simulink model "bfsk_demodulation_ber"  (R2021a)
settings: Solver=VariableStepAuto  StartTime=0.0  StopTime=2  RelTol=1e-3
libraries: dspsrcs4 x6, commfilt2 x5, commsink2 x2, commchan3 x1, commanapbnd3 x1, commrandsrc3 x1, simulink x1
settings Model: Creator=joycelai  LastModifiedBy=joycelai

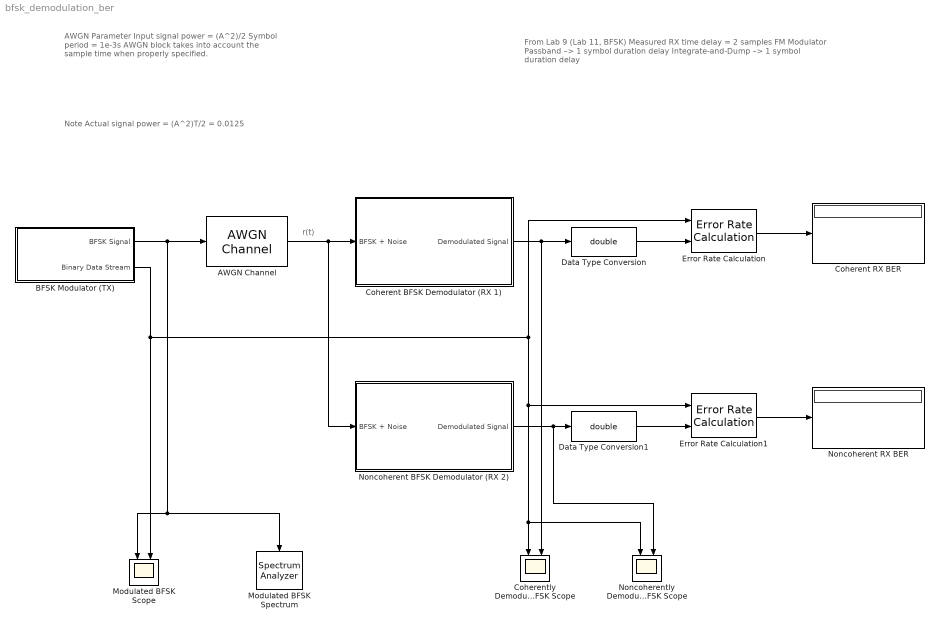
== system bfsk_demodulation_ber ==
  note: AWGN Parameter
      | Input signal power = (A^2)/2
      | Symbol period = 1e-3s
      |
      | AWGN block takes into account the
      | sample time when properly specified.
  note: r(t)
  note: Note
      | Actual signal power = (A^2)T/2 = 0.0125
  note: From Lab 9 (Lab 11, BFSK)
      | Measured RX time delay = 2 samples
      |
      | FM Modulator Passband –> 1 symbol duration delay
      | Integrate-and-Dump –> 1 symbol duration delay
  AWGN Channel : commchan3/AWGN Channel  InputProcessing=Columns as channels (frame based)  seed=67  noiseMode="Signal to noise ratio  (Eb/No)"  EbNodB=2  EsNodB=10  SNRdB=10  bitsPerSym=1  Ps=25/2  Tsym=1e-3  variance=1
  BFSK Modulator (TX) : Subsystem
  Coherent BFSK Demodulator (RX 1) : Subsystem
  Coherent RX BER : Display
      settings: Decimation=14
  Coherently Demodulated BFSK Scope : Scope  NumInputPorts=2
  Data Type Conversion : DataTypeConversion  OutDataTypeStr=double
  Data Type Conversion1 : DataTypeConversion  OutDataTypeStr=double
  Error Rate Calculation : commsink2/Error Rate Calculation  N=2  st_delay=0  cp_mode=Entire frame  subframe=[]  PMode=Port  WsName=ErrorVec  RsMode2=off  stop=off  numErr=100  maxBits=1e6
  Error Rate Calculation1 : commsink2/Error Rate Calculation  N=2  st_delay=0  cp_mode=Entire frame  subframe=[]  PMode=Port  WsName=ErrorVec  RsMode2=off  stop=off  numErr=100  maxBits=1e6
  Modulated BFSK Scope : Scope  NumInputPorts=2
  Modulated BFSK Spectrum : SpectrumAnalyzer
  Noncoherent BFSK Demodulator (RX 2) : Subsystem
  Noncoherent RX BER : Display
      settings: Decimation=14
  Noncoherently Demodulated BFSK Scope : Scope  NumInputPorts=2
  wires:
  Data Type Conversion/1 -> Error Rate Calculation/2
  BFSK Modulator (TX)/1(BFSK Signal) -> AWGN Channel/1, Modulated BFSK Spectrum/1, Modulated BFSK Scope/1
  Coherent BFSK Demodulator (RX 1)/1(Demodulated Signal) -> Data Type Conversion/1, Coherently Demodulated BFSK Scope/2
  BFSK Modulator (TX)/2(Binary Data Stream) -> Modulated BFSK Scope/2, Noncoherently Demodulated BFSK Scope/1, Coherently Demodulated BFSK Scope/1, Error Rate Calculation1/1, Error Rate Calculation/1
  Error Rate Calculation/1 -> Coherent RX BER/1
  AWGN Channel/1 -> Noncoherent BFSK Demodulator (RX 2)/1(BFSK + Noise), Coherent BFSK Demodulator (RX 1)/1(BFSK + Noise)
  Error Rate Calculation1/1 -> Noncoherent RX BER/1
  Data Type Conversion1/1 -> Error Rate Calculation1/2
  Noncoherent BFSK Demodulator (RX 2)/1(Demodulated Signal) -> Noncoherently Demodulated BFSK Scope/2, Data Type Conversion1/1

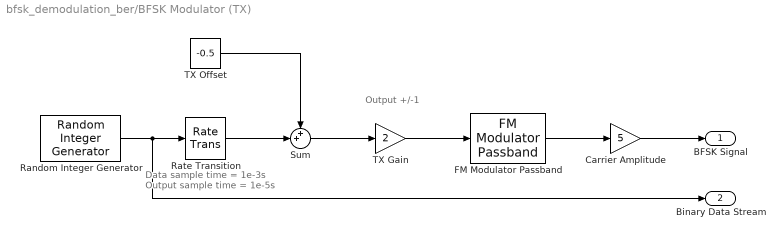
== system bfsk_demodulation_ber/BFSK Modulator (TX) ==
  note: Data sample time = 1e-3s
      | Output sample time = 1e-5s
  note: Output +/-1
  Carrier Amplitude : Gain  Gain=5
  FM Modulator Passband : commanapbnd3/FM Modulator Passband  Fc=10e3  Ph=pi/10  Kc=3e3
      settings: SourceProductBaseCode=CM
  Random Integer Generator : commrandsrc3/Random Integer Generator  SetSize=2  SeedSource=Auto  Seed=0  SampleTime=1e-3  SamplesPerFrame=1  OutputDataType=double  SimulateUsing=Interpreted execution
  Rate Transition : RateTransition  OutPortSampleTime=1e-5
  Sum : Sum  Inputs=++|
  TX Gain : Gain  Gain=2
  TX Offset : Constant  Value=-0.5
  BFSK Signal : Outport
  Binary Data Stream : Outport  Port=2
  wires:
  Random Integer Generator/1 -> Binary Data Stream/1, Rate Transition/1
  TX Gain/1 -> FM Modulator Passband/1
  Sum/1 -> TX Gain/1
  Carrier Amplitude/1 -> BFSK Signal/1
  FM Modulator Passband/1 -> Carrier Amplitude/1
  TX Offset/1 -> Sum/1
  Rate Transition/1 -> Sum/2

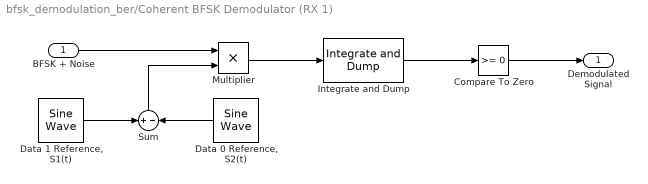
== system bfsk_demodulation_ber/Coherent BFSK Demodulator (RX 1) ==
  BFSK + Noise : Inport
  Compare To Zero : simulink/Logic and Bit Operations/Compare To Zero  relop=>=  OutDataTypeStr=uint8
  "Data 0 Reference, S2(t)" : dspsrcs4/Sine Wave  Amplitude=1  Frequency=(10e3)-(3e3)  Phase=pi/2+pi/10  SampleMode=Discrete  OutComplex=Real  CompMethod=Trigonometric fcn  TableSize=Speed  SampleTime=1e-5  SamplesPerFrame=1  ResetState=Restart at time zero  OutputFrames=off  dataType=double  wordLen=16  udDataType=sfix(16)  fracBitsMode=Best precision  numFracBits=15  OutDataTypeStr=double  LastOutDataTypeStr=double
  "Data 1 Reference, S1(t)" : dspsrcs4/Sine Wave  Amplitude=1  Frequency=(10e3)+(3e3)  Phase=pi/2+pi/10  SampleMode=Discrete  OutComplex=Real  CompMethod=Trigonometric fcn  TableSize=Speed  SampleTime=1e-5  SamplesPerFrame=1  ResetState=Restart at time zero  OutputFrames=off  dataType=double  wordLen=16  udDataType=sfix(16)  fracBitsMode=Best precision  numFracBits=15  OutDataTypeStr=double  LastOutDataTypeStr=double
  Integrate and Dump : commfilt2/Integrate and Dump  obssamples=100  offsetsamples=0  nodump=off  roundingMode=Floor  overflowMode=off  outputDataTypeStr=Inherit: Same as accumulator  outputLastDataTypeStr=Inherit: Same as accumulator
  Multiplier : Product
  Sum : Sum  Inputs=+|-
  Demodulated Signal : Outport  OutDataTypeStr=uint8
  wires:
  Multiplier/1 -> Integrate and Dump/1
  "Data 0 Reference, S2(t)"/1 -> Sum/2
  Sum/1 -> Multiplier/2
  BFSK + Noise/1 -> Multiplier/1
  "Data 1 Reference, S1(t)"/1 -> Sum/1
  Integrate and Dump/1 -> Compare To Zero/1
  Compare To Zero/1 -> Demodulated Signal/1

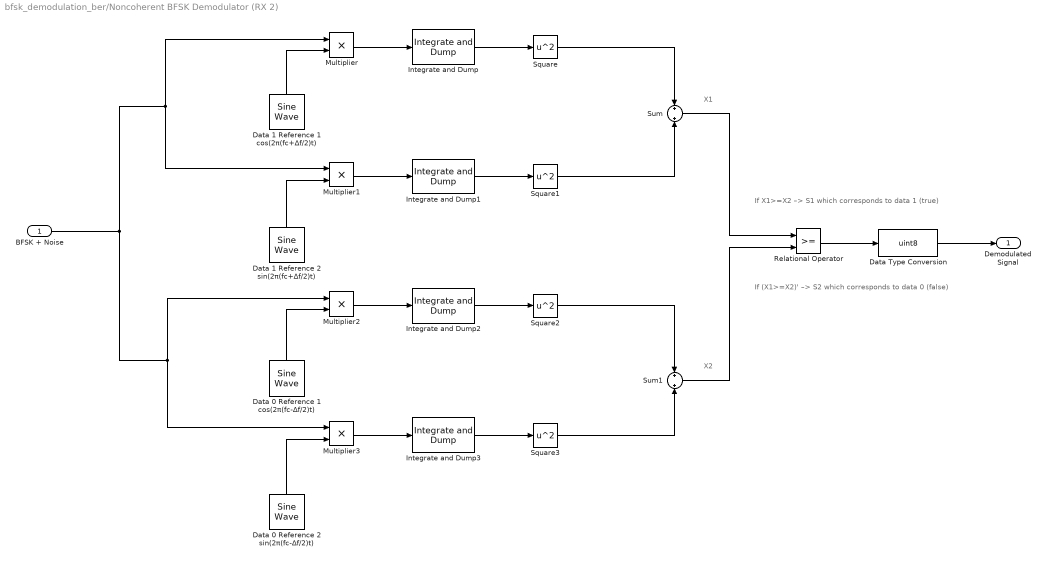
== system bfsk_demodulation_ber/Noncoherent BFSK Demodulator (RX 2) ==
  note: If (X1>=X2)' –> S2 which corresponds to data 0 (false)
  note: If X1>=X2 –> S1 which corresponds to data 1 (true)
  note: X2
  note: X1
  BFSK + Noise : Inport
  Data 0 Reference 1 cos(2π(fc-∆f/2)t) : dspsrcs4/Sine Wave  Amplitude=1  Frequency=(10e3)-(3e3)  Phase=pi/2  SampleMode=Discrete  OutComplex=Real  CompMethod=Trigonometric fcn  TableSize=Speed  SampleTime=1e-5  SamplesPerFrame=1  ResetState=Restart at time zero  OutputFrames=off  dataType=double  wordLen=16  udDataType=sfix(16)  fracBitsMode=Best precision  numFracBits=15  OutDataTypeStr=double  LastOutDataTypeStr=double
  Data 0 Reference 2 sin(2π(fc-∆f/2)t) : dspsrcs4/Sine Wave  Amplitude=1  Frequency=(10e3)-(3e3)  Phase=0  SampleMode=Discrete  OutComplex=Real  CompMethod=Trigonometric fcn  TableSize=Speed  SampleTime=1e-5  SamplesPerFrame=1  ResetState=Restart at time zero  OutputFrames=off  dataType=double  wordLen=16  udDataType=sfix(16)  fracBitsMode=Best precision  numFracBits=15  OutDataTypeStr=double  LastOutDataTypeStr=double
  Data 1 Reference 1 cos(2π(fc+∆f/2)t) : dspsrcs4/Sine Wave  Amplitude=1  Frequency=(10e3)+(3e3)  Phase=pi/2  SampleMode=Discrete  OutComplex=Real  CompMethod=Trigonometric fcn  TableSize=Speed  SampleTime=1e-5  SamplesPerFrame=1  ResetState=Restart at time zero  OutputFrames=off  dataType=double  wordLen=16  udDataType=sfix(16)  fracBitsMode=Best precision  numFracBits=15  OutDataTypeStr=double  LastOutDataTypeStr=double
  Data 1 Reference 2 sin(2π(fc+∆f/2)t) : dspsrcs4/Sine Wave  Amplitude=1  Frequency=(10e3)+(3e3)  Phase=0  SampleMode=Discrete  OutComplex=Real  CompMethod=Trigonometric fcn  TableSize=Speed  SampleTime=1e-5  SamplesPerFrame=1  ResetState=Restart at time zero  OutputFrames=off  dataType=double  wordLen=16  udDataType=sfix(16)  fracBitsMode=Best precision  numFracBits=15  OutDataTypeStr=double  LastOutDataTypeStr=double
  Data Type Conversion : DataTypeConversion  OutDataTypeStr=uint8
  Integrate and Dump{,1..3} (4 alike) : commfilt2/Integrate and Dump  obssamples=100  offsetsamples=0  nodump=off  roundingMode=Floor  overflowMode=off  outputDataTypeStr=Inherit: Same as accumulator  outputLastDataTypeStr=Inherit: Same as accumulator
  Multiplier{,1..3} (4 alike) : Product
  Relational Operator : RelationalOperator  RndMeth=Simplest
  Square{,1..3} (4 alike) : Math  Operator=square  SaturateOnIntegerOverflow=on
  Sum : Sum  Inputs=+||+
  Sum1 : Sum  Inputs=+||+
  Demodulated Signal : Outport  OutDataTypeStr=uint8
  wires:
  Multiplier/1 -> Integrate and Dump/1
  BFSK + Noise/1 -> Multiplier1/1, Multiplier/1, Multiplier2/1, Multiplier3/1
  Integrate and Dump/1 -> Square/1
  Multiplier1/1 -> Integrate and Dump1/1
  Integrate and Dump1/1 -> Square1/1
  Integrate and Dump2/1 -> Square2/1
  Multiplier2/1 -> Integrate and Dump2/1
  Integrate and Dump3/1 -> Square3/1
  Multiplier3/1 -> Integrate and Dump3/1
  Data 1 Reference 1 cos(2π(fc+∆f/2)t)/1 -> Multiplier/2
  Data 1 Reference 2 sin(2π(fc+∆f/2)t)/1 -> Multiplier1/2
  Data 0 Reference 1 cos(2π(fc-∆f/2)t)/1 -> Multiplier2/2
  Data 0 Reference 2 sin(2π(fc-∆f/2)t)/1 -> Multiplier3/2
  Square/1 -> Sum/1
  Square1/1 -> Sum/2
  Square2/1 -> Sum1/1
  Square3/1 -> Sum1/2
  Sum/1 -> Relational Operator/1
  Sum1/1 -> Relational Operator/2
  Relational Operator/1 -> Data Type Conversion/1
  Data Type Conversion/1 -> Demodulated Signal/1
